simulink model "no_state_tekitou"  (R2014a)
settings: Solver=FixedStepDiscrete  StartTime=0.0  StopTime=10.0  FixedStep=0.1  RelTol=1e-3
settings Model: Creator=yoshi12  LastModifiedBy=yoshi12

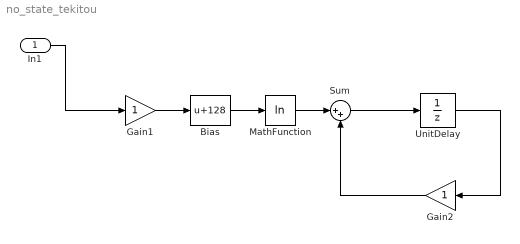
== system no_state_tekitou ==
  In1 : Inport
  Bias : Bias  Bias=128
  Gain1 : Gain
  Gain2 : Gain
  MathFunction : Math  Operator=log  SaturateOnIntegerOverflow=on
  Sum : Sum  Inputs=|++
  UnitDelay : UnitDelay  SampleTime=-1
  wires:
  Sum/1 -> UnitDelay/1
  UnitDelay/1 -> Gain2/1
  In1/1 -> Gain1/1
  Gain1/1 -> Bias/1
  Bias/1 -> MathFunction/1
  Gain2/1 -> Sum/2
  MathFunction/1 -> Sum/1
